simulink model "example3"  (R2024a)
settings: Solver=VariableStepAuto  StartTime=0.0  StopTime=10.0  RelTol=1e-3
libraries: simulink x2
settings Model: Creator=guirl  LastModifiedBy=guirl

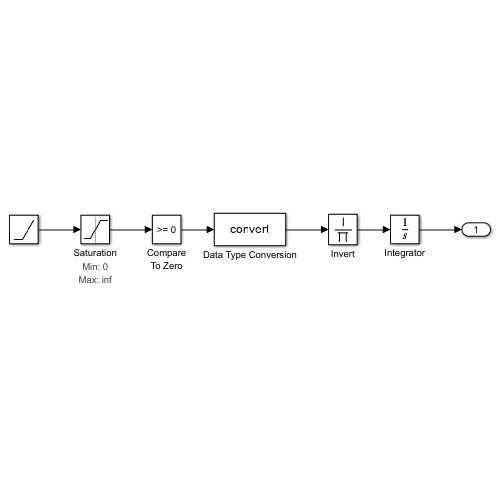
[thumbnail: Simulink's stored preview of the top-level diagram]
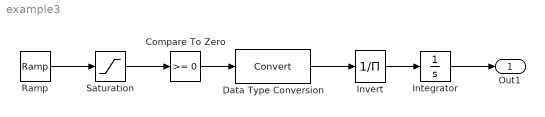
== system example3 ==
  Compare To Zero : simulink/Logic and Bit Operations/Compare To Constant  relop=>=  const=0  OutDataTypeStr=boolean  ZeroCross=off
  Data Type Conversion : DataTypeConversion  SaturateOnIntegerOverflow=off  RndMeth=Floor
  Integrator : Integrator
  Invert : Product  Inputs=/
  Ramp : simulink/Sources/Ramp  slope=-1.123  start=0  InitialOutput=1
  Saturation : Saturate  UpperLimit=inf  LowerLimit=0
      settings: AttributesFormatString=|
      | Min: %<LowerLimit>
      | Max: %<UpperLimit>
  Out1 : Outport
  wires:
  Ramp/1 -> Saturation/1
  Saturation/1 -> Compare To Zero/1
  Compare To Zero/1 -> Data Type Conversion/1
  Invert/1 -> Integrator/1
  Integrator/1 -> Out1/1
  Data Type Conversion/1 -> Invert/1
